simulink model "Brown_Full_Sim"  (R2025b)
settings: Solver=VariableStepAuto  StartTime=0.0  StopTime=10.0  RelTol=1e-3
values from neighbouring files (symbols this model uses):
  eul_init = scenario.eul_init    [Brown_6DOF_Init_main.m]    (also in Full_Sim_Init.m; Init_Main.m = deg2rad([0; 0; 0]); Run_Main.m = runSpec.eul_init)
  g = scenario.g    [Brown_6DOF_Init_main.m]    (also in Full_Sim_Init.m; Init_Main.m = 9.81; aircraft_def.m = value)
  J = aircraft.J    [Brown_6DOF_Init_main.m]    (also in Full_Sim_Init.m; HOMEWORK7_trim_linmod_live_source.m = zeros(4,3); Init_Main.m; aircraft_def.m = I_total)
  Motor_RPMs = localGroupMotorRPMs(Motor_RPMs_legacy)    [Brown_6DOF_Init_main.m]    (also in Full_Sim_Init.m = scenario.Motor_RPMs; Init_Main.m = motor_rpm_value * ones(4, 1); Run_Main.m = runSpec.Motor_RPMs)
  omega_init = scenario.omega_init    [Brown_6DOF_Init_main.m]    (also in Full_Sim_Init.m; Init_Main.m = [0.0; 0.0; 0.0]; Run_Main.m = runSpec.omega_init)
  pos_init = scenario.pos_init    [Brown_6DOF_Init_main.m]    (also in Full_Sim_Init.m; Init_Main.m = pos_init(:); Run_Main.m = runSpec.pos_init)
  q = q / norm(q)    [HOMEWORK7_trim_linmod_live_source.m]    (also in attitude_complementary_step.m = gyro_meas(2))
  r = positions(i, :).'-cg(:)    [Run_INDI_Qdot_Effectiveness_Audit.m]    (also in attitude_complementary_step.m = gyro_meas(3))
  Tilt_angles = localCollapseFrontTiltAngles(Tilt_angles_legacy)    [Brown_6DOF_Init_main.m]    (also in Full_Sim_Init.m = scenario.Tilt_angles; Init_Main.m = tilt_angle_deg * ones(2, 1); Run_Main.m = runSpec.Tilt_angles)
  V_init = scenario.V_init    [Brown_6DOF_Init_main.m]    (also in Full_Sim_Init.m; Init_Main.m = [75.0; 0.0; 0.0]; Run_Main.m = runSpec.V_init)
undefined symbols (not defined in the file or in its folder): F, Light, magnitude, MIL
libraries: Brown_Flight_Controls_lib x13, aerolibfltsims x1, aerolibwind2 x1
settings Model: Creator=zbrown  LastModifiedBy=zbrown

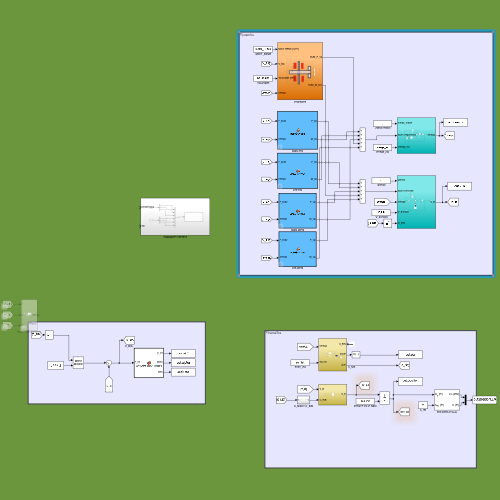
[thumbnail: Simulink's stored preview of the top-level diagram]
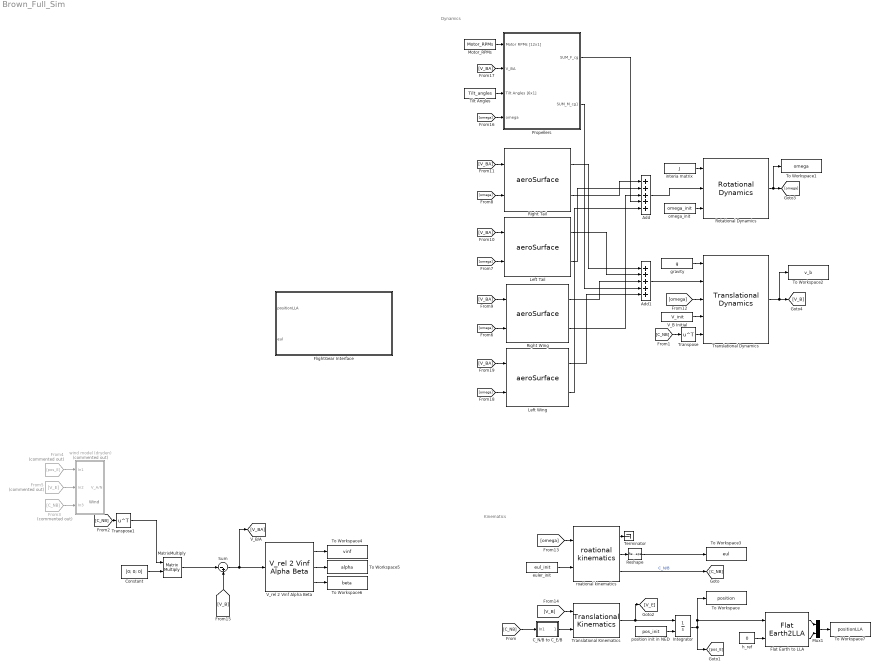
== system Brown_Full_Sim ==
  note: Wind
  note: Dynamics
  note: Kinematics
  " Motor_RPMs" : Constant  Value=Motor_RPMs
  " Tilt Angles" : Constant  Value=Tilt_angles
  " V_B Initial" : Constant  Value=V_init
  " gravity" : Constant  Value=g
  " interia matrix" : Constant  Value=J
  Add : Sum  Inputs=+++++
  Add1 : Sum  Inputs=+++++
  C_N/B to C_E/B : Subsystem
  Constant : Constant  Value=[0; 0; 0]
  Flat Earth to LLA : FlatEarth2LLA
  FlightGear Interface : Subsystem
  From3 : From  Commented=on  GotoTag=C_NB
  From4 : From  Commented=on  GotoTag=pos_E
  From5 : From  Commented=on  GotoTag=V_E
  Integrator : Integrator  InitialConditionSource=external
  Left Tail : Brown_Flight_Controls_lib/aeroSurface  surf=tailL  CG=CG
  Left Wing : Brown_Flight_Controls_lib/aeroSurface  surf=wingL  CG=CG
  MatrixMultiply : Product  Multiplication=Matrix(*)
  Mux1 : Mux  Inputs=2
  Propellers : Subsystem
  Reshape : Reshape
  Right Tail : Brown_Flight_Controls_lib/aeroSurface  surf=tailR  CG=CG
  Right Wing : Brown_Flight_Controls_lib/aeroSurface  surf=wingR  CG=CG
  Rotational Dynamics : Brown_Flight_Controls_lib/Rotational Dynamics  SystemSampleTime=-1  VariantActivationTime=update diagram  EmptyChoice=off  PassThrough=off  PassThroughVariantControl=(default)  EmptyChoiceVariantControl=(default)  AllowFlexibleInterface=on  Latency=0  AutoFrameSizeCalculation=off
  Sum : Sum  Inputs=|-+
  Terminator : Terminator
  To Workspace : ToWorkspace  VariableName=position  SaveFormat=Timeseries  SampleTime=-1
  To Workspace1 : ToWorkspace  VariableName=omega  SaveFormat=Timeseries  SampleTime=-1
  To Workspace2 : ToWorkspace  VariableName=v_b  SaveFormat=Timeseries  SampleTime=-1
  To Workspace3 : ToWorkspace  VariableName=eul  SaveFormat=Timeseries  SampleTime=-1
  To Workspace4 : ToWorkspace  VariableName=vinf  SaveFormat=Timeseries  SampleTime=-1
  To Workspace5 : ToWorkspace  VariableName=alpha  SaveFormat=Timeseries  SampleTime=-1
  To Workspace6 : ToWorkspace  VariableName=beta  SaveFormat=Timeseries  SampleTime=-1
  To Workspace7 : ToWorkspace  VariableName=positionLLA  SaveFormat=Timeseries  SampleTime=-1
  Translational Dynamics : Brown_Flight_Controls_lib/Translational Dynamics  SystemSampleTime=-1  VariantActivationTime=update diagram  EmptyChoice=off  PassThrough=off  PassThroughVariantControl=(default)  EmptyChoiceVariantControl=(default)  AllowFlexibleInterface=on  Latency=0  AutoFrameSizeCalculation=off
  Translational Kinematics : Brown_Flight_Controls_lib/Translational Kinematics  SystemSampleTime=-1  VariantActivationTime=update diagram  EmptyChoice=off  PassThrough=off  PassThroughVariantControl=(default)  EmptyChoiceVariantControl=(default)  AllowFlexibleInterface=on  Latency=0  AutoFrameSizeCalculation=off
  Transpose : Math  Operator=transpose
  Transpose1 : Math  Operator=transpose
  V_rel 2 Vinf Alpha Beta : Brown_Flight_Controls_lib/V_rel 2 Vinf Alpha Beta  SystemSampleTime=-1  VariantActivationTime=update diagram  EmptyChoice=off  PassThrough=off  PassThroughVariantControl=(default)  EmptyChoiceVariantControl=(default)  AllowFlexibleInterface=on  Latency=0  AutoFrameSizeCalculation=off
  euler_init : Constant  Value=eul_init
  h_ref : Constant  Value=0
  omega_init : Constant  Value=omega_init
  position init in NED : Constant  Value=pos_init
  roational kinematics : Brown_Flight_Controls_lib/roational kinematics  SystemSampleTime=-1  VariantActivationTime=update diagram  EmptyChoice=off  PassThrough=off  PassThroughVariantControl=(default)  EmptyChoiceVariantControl=(default)  AllowFlexibleInterface=on  Latency=0  AutoFrameSizeCalculation=off
  wind model (dryden) : Subsystem  Commented=on
  wires:
  Transpose/1 -> Translational Dynamics/5
  roational kinematics/3 -> [C_NB]  "C_N/B"
  roational kinematics/1 -> Terminator/1
  roational kinematics/2 -> Reshape/1
  Rotational Dynamics/1 -> [omega], To Workspace1/1
  Translational Dynamics/1 -> [V_B], To Workspace2/1
  Translational Kinematics/1 -> [V_E], Integrator/1
  position init in NED/1 -> Integrator/2
  Integrator/1 -> Flat Earth to LLA/1, To Workspace/1, [pos_E]
  euler_init/1 -> roational kinematics/2
  omega_init/1 -> Rotational Dynamics/3
  Add/1 -> Rotational Dynamics/2
  " interia matrix"/1 -> Rotational Dynamics/1
  " gravity"/1 -> Translational Dynamics/1
  Add1/1 -> Translational Dynamics/2
  " V_B Initial"/1 -> Translational Dynamics/4
  Reshape/1 -> To Workspace3/1
  C_N/B to C_E/B/1(Out1) -> Translational Kinematics/2
  [C_NB] -> C_N/B to C_E/B/1(In1)
  [C_NB] -> Transpose/1
  MatrixMultiply/1 -> Sum/1
  Transpose1/1 -> MatrixMultiply/1
  [C_NB] -> Transpose1/1
  Sum/1 -> [V_BA], V_rel 2 Vinf Alpha Beta/1
  From4/1 -> wind model (dryden)/1(In1)
  From5/1 -> wind model (dryden)/2(In2)
  From3/1 -> wind model (dryden)/3(In3)
  [omega] -> Right Wing/2
  [omega] -> Left Tail/2
  [V_BA] -> Right Wing/1
  [V_BA] -> Left Tail/1
  [V_BA] -> Right Tail/1
  V_rel 2 Vinf Alpha Beta/1 -> To Workspace4/1
  V_rel 2 Vinf Alpha Beta/2 -> To Workspace5/1
  V_rel 2 Vinf Alpha Beta/3 -> To Workspace6/1
  [omega] -> Translational Dynamics/3
  [omega] -> roational kinematics/1
  [V_B] -> Translational Kinematics/1
  Right Wing/1 -> Add1/3
  Left Tail/1 -> Add1/2
  Right Tail/1 -> Add1/1
  Right Tail/2 -> Add/1
  Left Tail/2 -> Add/2
  Right Wing/2 -> Add/3
  [V_B] -> Sum/2
  [omega] -> Right Tail/2
  " Tilt Angles"/1 -> Propellers/3(Tilt Angles [6x1])
  [omega] -> Propellers/4(omega)
  [V_BA] -> Propellers/2(V_BA)
  " Motor_RPMs"/1 -> Propellers/1(Motor RPMs [12x1])
  Propellers/1(SUM_F_cg) -> Add/4
  Propellers/2(SUM_M_cg1) -> Add1/4
  h_ref/1 -> Flat Earth to LLA/2
  Mux1/1 -> To Workspace7/1
  Flat Earth to LLA/1 -> Mux1/1
  Flat Earth to LLA/2 -> Mux1/2
  Constant/1 -> MatrixMultiply/2
  [omega] -> Left Wing/2
  [V_BA] -> Left Wing/1
  Left Wing/2 -> Add/5
  Left Wing/1 -> Add1/5

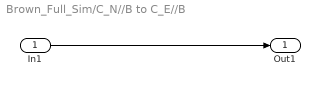
== system Brown_Full_Sim/C_N//B to C_E//B ==
  In1 : Inport
  Out1 : Outport
  wires:
  In1/1 -> Out1/1

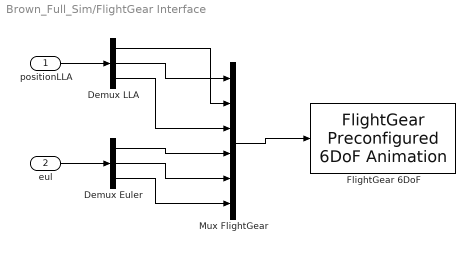
== system Brown_Full_Sim/FlightGear Interface ==
  positionLLA : Inport
  eul : Inport  Port=2
  Demux Euler : Demux  Outputs=3
  Demux LLA : Demux  Outputs=3
  FlightGear 6DoF : aerolibfltsims/FlightGear Preconfigured 6DoF Animation  xFlightGearVersion=v2019.1  DestinationIpAddress=127.0.0.1  DestinationPort=5502  SampleTime=1/30  packetVersion=24
  Mux FlightGear : Mux  Inputs=6
  wires:
  positionLLA/1 -> Demux LLA/1
  eul/1 -> Demux Euler/1
  Demux LLA/2 -> Mux FlightGear/1
  Demux LLA/1 -> Mux FlightGear/2
  Demux LLA/3 -> Mux FlightGear/3
  Demux Euler/1 -> Mux FlightGear/4
  Demux Euler/2 -> Mux FlightGear/5
  Demux Euler/3 -> Mux FlightGear/6
  Mux FlightGear/1 -> FlightGear 6DoF/1

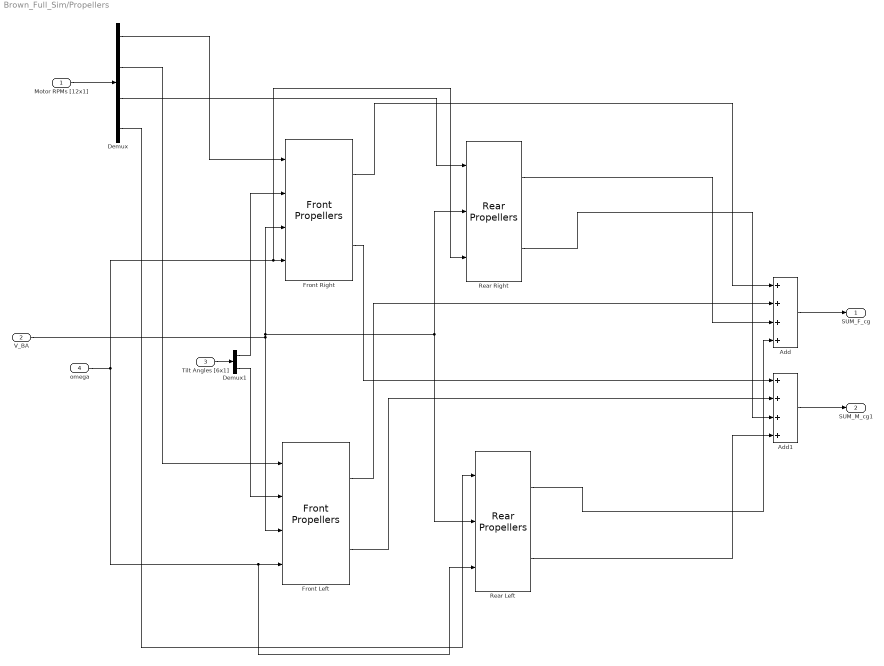
== system Brown_Full_Sim/Propellers ==
  Motor RPMs [12x1] : Inport
  V_BA : Inport  Port=2
  Tilt Angles [6x1] : Inport  Port=3
  omega : Inport  Port=4
  Add : Sum  Inputs=++++
  Add1 : Sum  Inputs=++++
  Demux : Demux
  Demux1 : Demux  Outputs=2
  Front Left : Brown_Flight_Controls_lib/Front Propellers  pivot_pos=prop.posFL  hub_offset=prop.hub_offset  kT=prop.k_Thrust  kQ=prop.k_Torque  CG=CG  spin_dir=prop.Lspin_dir
  Front Right : Brown_Flight_Controls_lib/Front Propellers  pivot_pos=prop.posFR  hub_offset=prop.hub_offset  kT=prop.k_Thrust  kQ=prop.k_Torque  CG=CG  spin_dir=prop.Rspin_dir
  Rear Left : Brown_Flight_Controls_lib/Rear Propellers  prop_pos=prop.posRL  kT=prop.k_Thrust  kQ=prop.k_Torque  CG=CG  spin_dir=prop.Lspin_dir
  Rear Right : Brown_Flight_Controls_lib/Rear Propellers  prop_pos=prop.posRR  kT=prop.k_Thrust  kQ=prop.k_Torque  CG=CG  spin_dir=prop.Rspin_dir
  SUM_F_cg : Outport
  SUM_M_cg1 : Outport  Port=2
  wires:
  V_BA/1 -> Front Right/3, Rear Left/2, Rear Right/2, Front Left/3
  Add/1 -> SUM_F_cg/1
  Add1/1 -> SUM_M_cg1/1
  Motor RPMs [12x1]/1 -> Demux/1
  Demux/1 -> Front Right/1
  Demux/2 -> Front Left/1
  Demux/3 -> Rear Right/1
  Demux/4 -> Rear Left/1
  Tilt Angles [6x1]/1 -> Demux1/1
  Demux1/1 -> Front Right/2
  Demux1/2 -> Front Left/2
  omega/1 -> Rear Right/3, Front Right/4, Rear Left/3, Front Left/4
  Front Right/1 -> Add/1
  Rear Right/1 -> Add/3
  Front Left/1 -> Add/2
  Rear Left/1 -> Add/4
  Front Right/2 -> Add1/1
  Rear Right/2 -> Add1/3
  Front Left/2 -> Add1/2
  Rear Left/2 -> Add1/4

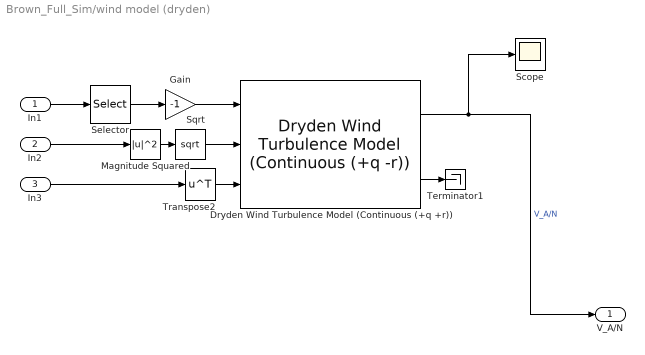
== system Brown_Full_Sim/wind model (dryden) ==
  In1 : Inport
  In2 : Inport  Port=2
  In3 : Inport  Port=3
  Dryden Wind Turbulence Model (Continuous (+q +r)) : aerolibwind2/Dryden Wind Turbulence Model  (Continuous (+q -r))  units=Metric (MKS)  spec=MIL-F-8785C  model=Continuous Dryden (+q +r)  W20=15  Wdeg=0  TurbProb=10^-2 - Light  L_high=533.4  Wingspan=10  ts=0.1  Seed=[23341 23342 23343 23344]  T_on=on
      settings: LibrarySourceBlock=|
      | aerolibwind2/Dryden Wind Turbulence Model
      | (Continuous (+q +r))
  Gain : Gain  Gain=-1
  Magnitude Squared : Math  Operator=magnitude^2
  Scope : Scope
  Selector : Selector  InputPortWidth=3  IndexOptions=Index vector (dialog)  Indices=[3]  OutputSizes=1
  Sqrt : Sqrt
  Terminator1 : Terminator
  Transpose2 : Math  Operator=transpose
  V_A/N : Outport
  wires:
  In1/1 -> Selector/1
  Sqrt/1 -> Dryden Wind Turbulence Model (Continuous (+q +r))/2
  Dryden Wind Turbulence Model (Continuous (+q +r))/1 -> V_A/N/1, Scope/1  "V_A/N"
  In3/1 -> Transpose2/1
  Transpose2/1 -> Dryden Wind Turbulence Model (Continuous (+q +r))/3
  In2/1 -> Magnitude Squared/1
  Dryden Wind Turbulence Model (Continuous (+q +r))/2 -> Terminator1/1
  Gain/1 -> Dryden Wind Turbulence Model (Continuous (+q +r))/1
  Selector/1 -> Gain/1
  Magnitude Squared/1 -> Sqrt/1
